simulink model "Sim_Test_PID_MPC"  (R2023b)
settings: Solver=ode4  StartTime=0.0  StopTime=Sim_time  FixedStep=dt  RelTol=1e-3
values from neighbouring files (symbols this model uses):
  den = [1 5.235 5.375 0]    [Run_Sim_PID_MPC.m]
  den_u = 1;[1 12 225]    [Run_Sim_PID_MPC.m]
  dist_amp = 2    [Run_Sim_PID_MPC.m]
  dt = 0.01    [Run_Sim_PID_MPC.m]
  Dtest = 0    [Run_Sim_PID_MPC.m]
  Kaw = 0    [Run_Sim_PID_MPC.m]
  Kd = 4    [Run_Sim_PID_MPC.m]
  Ki = 0.0    (= 0)    [Run_Sim_PID_MPC.m]
  Kp = 6    [Run_Sim_PID_MPC.m]
  Ktest = 1    [Run_Sim_PID_MPC.m]
  noise_var = 0.0025    [Run_Sim_PID_MPC.m]
  num = [1.816 5.737]    [Run_Sim_PID_MPC.m]
  num_u = 1;225    [Run_Sim_PID_MPC.m]
  RSat = inf    [Run_Sim_PID_MPC.m]
  Sat = inf    [Run_Sim_PID_MPC.m]
  Set_Amp = 1    [Run_Sim_PID_MPC.m]
libraries: mpclib x1
settings Model: Creator=3056709  LastModifiedBy=ps22aae
settings DebuggingCC: UnconnectedInputMsg=warning  UnconnectedOutputMsg=warning  UnconnectedLineMsg=warning
settings ModelReferenceCC: EnableRefExpFcnMdlSchedulingChecks=on
settings RTWCC: DLArmComputeVersion=19.05

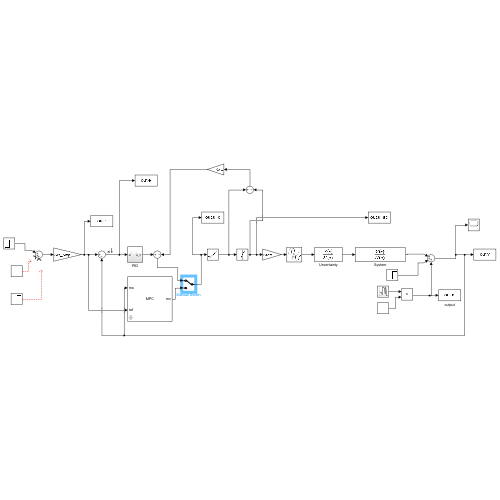
[thumbnail: Simulink's stored preview of the top-level diagram]
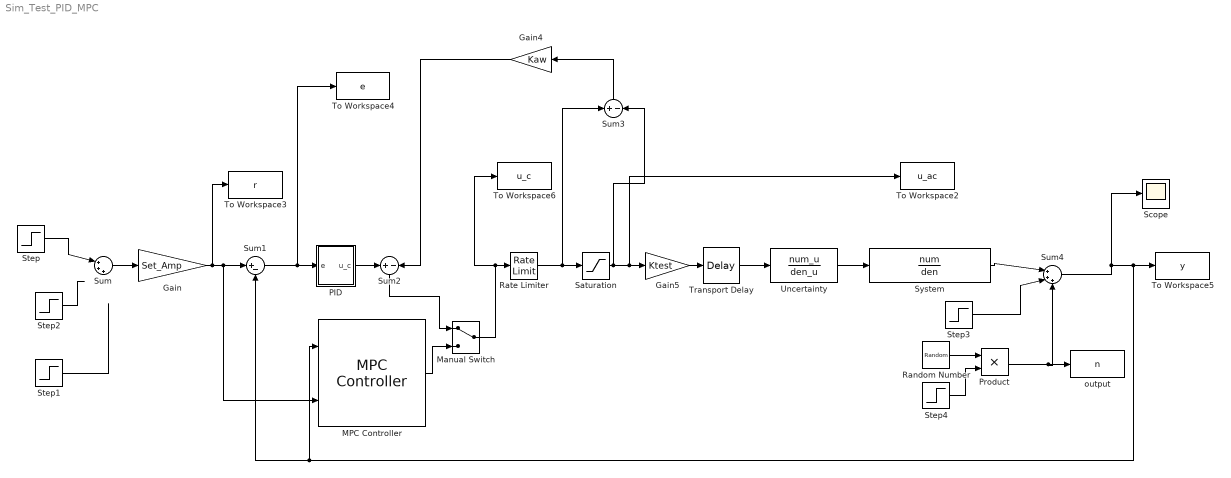
== system Sim_Test_PID_MPC ==
  Gain : Gain  Gain=Set_Amp
  Gain4 : Gain  Gain=Kaw
  Gain5 : Gain  Gain=Ktest
  MPC Controller : mpclib/MPC Controller  SCDEnableBlockLinearizationSpecification=on  mpcobj=mpc1  is_multiple=0  enable_value=0  return_u0=off  updateMPCinCallerWorkspace=on  md_inport=off  mv_inport=off  uref_inport=off  return_cost=off  return_mvseq=off  return_qpstatus=off  return_xseq=off  return_state=off  return_ovseq=off  state_inport=off  umin_inport=off  umax_inport=off  ymin_inport=off  ymax_inport=off  cc_inport=off  ywt_inport=off  uwt_inport=off  duwt_inport=off  rhoeps_inport=off  pm_inport=off  MaximumP=10  HorizonChoice=FixedHorizon  n_ts=0.01  n_p=120  n_mv=1  n_md=0  n_ud=0  n_mo=1  n_uo=0  BlockDataType=double  SampleTimeInherited=off  switch_inport=off
  Manual Switch : ManualSwitch
  PID : Subsystem
  Product : Product
  Random Number : RandomNumber  Variance=noise_var  SampleTime=dt
  Rate Limiter : RateLimiter  RisingSlewLimit=RSat  FallingSlewLimit=-RSat  SampleTimeMode=inherited
  Saturation : Saturate  UpperLimit=Sat  LowerLimit=-Sat
  Scope : Scope
  Step : Step  Time=0  SampleTime=0
  Step1 : Step  Time=40  After=3  SampleTime=0
  Step2 : Step  Time=21  After=-2  SampleTime=0
  Step3 : Step  Time=15  After=dist_amp  SampleTime=0
  Step4 : Step  Time=20  SampleTime=0
  Sum : Sum  Inputs=|+++
  Sum1 : Sum  Inputs=|+-
  Sum2 : Sum  Inputs=+-
  Sum3 : Sum  Inputs=+-
  Sum4 : Sum  Inputs=|+++
  System : TransferFcn  Numerator=num  Denominator=den
  To Workspace2 : ToWorkspace  VariableName=u_ac  SampleTime=-1
  To Workspace3 : ToWorkspace  VariableName=r  SampleTime=-1
  To Workspace4 : ToWorkspace  VariableName=e  SampleTime=-1
  To Workspace5 : ToWorkspace  VariableName=y  SampleTime=-1
  To Workspace6 : ToWorkspace  VariableName=u_c  SampleTime=-1
  Transport Delay : TransportDelay  DelayTime=Dtest
  Uncertainty : TransferFcn  Numerator=num_u  Denominator=den_u
  output : ToWorkspace  VariableName=n  SampleTime=-1
  wires:
  Sum4/1 -> To Workspace5/1, MPC Controller/1, Sum1/2, Scope/1
  Sum1/1 -> To Workspace4/1, PID/1(e)
  Sum/1 -> Gain/1
  Manual Switch/1 -> To Workspace6/1, Rate Limiter/1
  Transport Delay/1 -> Uncertainty/1
  Gain/1 -> MPC Controller/2, Sum1/1, To Workspace3/1
  Gain5/1 -> Transport Delay/1
  Uncertainty/1 -> System/1
  Step/1 -> Sum/1
  Step2/1 -> ?
  Step1/1 -> ?
  MPC Controller/1 -> Manual Switch/2
  PID/1(u_c) -> Sum2/1
  Saturation/1 -> To Workspace2/1, Gain5/1, Sum3/2
  Sum3/1 -> Gain4/1
  Rate Limiter/1 -> Saturation/1, Sum3/1
  Gain4/1 -> Sum2/2
  Sum2/1 -> Manual Switch/1
  Step4/1 -> Product/2
  Random Number/1 -> Product/1
  Step3/1 -> Sum4/2
  Product/1 -> Sum4/3, output/1
  System/1 -> Sum4/1

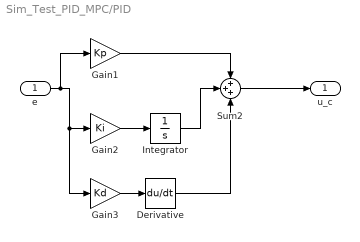
== system Sim_Test_PID_MPC/PID ==
  e : Inport
  Derivative : Derivative
  Gain1 : Gain  Gain=Kp
  Gain2 : Gain  Gain=Ki
  Gain3 : Gain  Gain=Kd
  Integrator : Integrator
  Sum2 : Sum  Inputs=+++
  u_c : Outport
  wires:
  Gain2/1 -> Integrator/1
  Sum2/1 -> u_c/1
  Gain3/1 -> Derivative/1
  Integrator/1 -> Sum2/2
  Derivative/1 -> Sum2/3
  Gain1/1 -> Sum2/1
  e/1 -> Gain1/1, Gain3/1, Gain2/1
